simulink model "Prop_VV_jonny"  (R2020b)
settings: Solver=VariableStepAuto  StartTime=0.0  StopTime=10.0  RelTol=1e-3
settings Model: Creator=Jonathan van Zyl  LastModifiedBy=Jonathan van Zyl

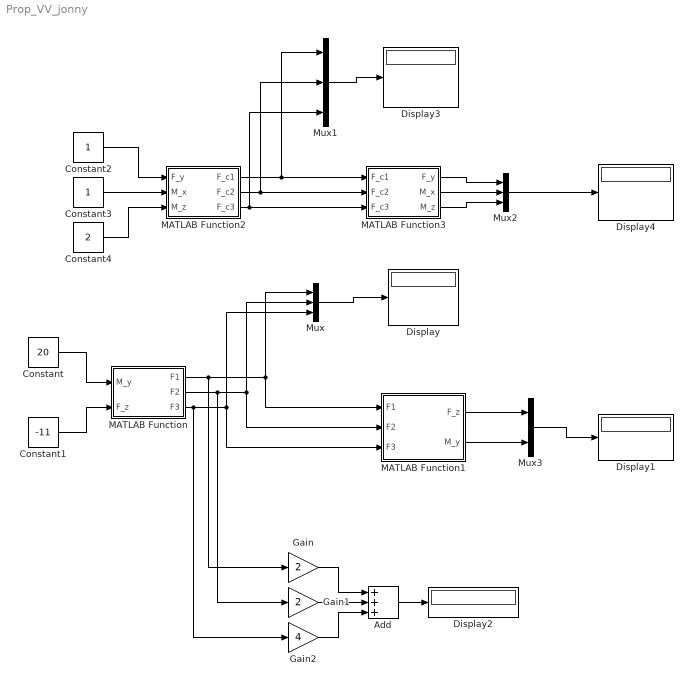
== system Prop_VV_jonny ==
  Add : Sum  Inputs=+++
  Constant : Constant  Value=20
  Constant1 : Constant  Value=-11
  Constant2 : Constant
  Constant3 : Constant
  Constant4 : Constant  Value=2
  Display{,1..4} (5 alike) : Display
  Gain : Gain  Gain=2
  Gain1 : Gain  Gain=2
  Gain2 : Gain  Gain=4
  MATLAB Function : MATLAB Function  TreatAsAtomicUnit=on
  MATLAB Function1 : MATLAB Function  TreatAsAtomicUnit=on
  MATLAB Function2 : MATLAB Function  TreatAsAtomicUnit=on
  MATLAB Function3 : MATLAB Function  TreatAsAtomicUnit=on
  Mux : Mux  Inputs=3
  Mux1 : Mux  Inputs=3
  Mux2 : Mux  Inputs=3
  Mux3 : Mux  Inputs=2
  wires:
  Constant/1 -> MATLAB Function/1(M_y)
  Constant1/1 -> MATLAB Function/2(F_z)
  MATLAB Function/1(F1) -> Gain/1, MATLAB Function1/1(F1), Mux/1
  MATLAB Function/2(F2) -> Gain1/1, MATLAB Function1/2(F2), Mux/2
  MATLAB Function/3(F3) -> Gain2/1, MATLAB Function1/3(F3), Mux/3
  Mux/1 -> Display/1
  Constant2/1 -> MATLAB Function2/1(F_y)
  Constant3/1 -> MATLAB Function2/2(M_x)
  Constant4/1 -> MATLAB Function2/3(M_z)
  MATLAB Function2/1(F_c1) -> MATLAB Function3/1(F_c1), Mux1/1
  MATLAB Function2/2(F_c2) -> MATLAB Function3/2(F_c2), Mux1/2
  MATLAB Function2/3(F_c3) -> Mux1/3, MATLAB Function3/3(F_c3)
  Mux1/1 -> Display3/1
  MATLAB Function3/1(F_y) -> Mux2/1
  MATLAB Function3/3(M_z) -> Mux2/3
  MATLAB Function3/2(M_x) -> Mux2/2
  Mux2/1 -> Display4/1
  MATLAB Function1/1(F_z) -> Mux3/1
  MATLAB Function1/2(M_y) -> Mux3/2
  Mux3/1 -> Display1/1
  Gain/1 -> Add/1
  Gain1/1 -> Add/2
  Gain2/1 -> Add/3
  Add/1 -> Display2/1

== matlab function Prop_VV_jonny/MATLAB Function1 ==
  data: F1 input; F_z output; F2 input; M_y output; F3 input
function [F_z, M_y] = fcn(F1, F2, F3)
xt_1 = 1.2598;
xb_1 = 2.2598;
xt_3 = -1.3402;
x_t1 = xt_1;
x_b1 = xb_1;
x_t3 = xt_3;

M_y = -100;
F_z = 0;

A_mat = [1 1;
    xt_1 xb_1];

A_inv = inv(A_mat);

force = [F1; F2];

back = A_mat*force;
backtrack = [4*F3; 4*F3*xt_3];
forceback = back+backtrack;
F_z = forceback(1);
M_y = forceback(2);
end

== matlab function Prop_VV_jonny/MATLAB Function ==
  data: M_y input; F1 output; F_z input; F2 output; F3 output
function [F1, F2, F3] = fcn(M_y, F_z)
xt_1 = 1.2598;
xb_1 = 2.2598;
xt_3 = -1.3402;
x_t1 = xt_1;
x_b1 = xb_1;
x_t3 = xt_3;



A_mat = [1 1;
    xt_1 xb_1];

A_inv = inv(A_mat);

p_0 = 0.2;
p_minus1 = 0;
step = 1000;
Converged = 0;
p_list = [];
x_list = [];
y_list = [];
J_list = [];
Fzz =[];
Myy =[];
while Converged == 0
    B = [(F_z - 4*p_0); (M_y - 4*p_0*xt_3)];
    force_0 = (A_inv*B);
    J_0 = sqrt(force_0(1)^2 + force_0(2)^2 + p_0^2);
    back = A_mat*force_0;
    backtrack = [4*p_0; 4*p_0*xt_3];
    forceback = back+backtrack;
    diff = sum(abs(forceback - [F_z; M_y]));
    if diff > 10^(-7)
        disp('Error')
        break
    end
    force = force_0;
    J = J_0;
    p = p_0;
    
    p_1 = p_0 + step;
    B = [(F_z - 4*p_1); (M_y - 4*p_1*xt_3)];
    force_1 = (A_inv*B);
    J_1 = sqrt(force_1(1)^2 + force_1(2)^2 + p_1^2);
    back = A_mat*force_1;
    backtrack = [4*p_1; 4*p_1*xt_3];
    forceback = back+backtrack;
    diff = sum(abs(forceback - [F_z; M_y]));
    if diff > 10^(-7)
        disp('Error')
        break
    end
    if J_1 < J_0
        force = force_1;
        J = J_1;
        p = p_1;
    end
    
    p_2 = p_0 - step;
    B = [(F_z - 4*p_2); (M_y - 4*p_2*xt_3)];
    force_2 = (A_inv*B);
    J_2 = sqrt(force_2(1)^2 + force_2(2)^2 + p_2^2);
    back = A_mat*force_2;
    backtrack = [4*p_2; 4*p_2*xt_3];
    forceback = back+backtrack;
    diff = sum(abs(forceback - [F_z; M_y]));
    if diff > 10^(-7)
        disp('Error')
        break
    end
    if J_2 < J_0 && J_2 < J_1
        force = force_2;
        J = J_2;
        p = p_2;
    end
    
    if p_minus1 < p_0 && p_0 < p
        step = step;
    elseif p_minus1 > p_0 && p_0 > p
        step = step;
    else
        step = step*0.9;
    end
        
    p_minus1 = p_0;
    p_0 = p;
    p_list = [p_list; p_0];
    x_list = [x_list; force(1)];
    y_list = [y_list; force(2)];
    J_list = [J_list; J];
    if step < abs(min([F_z,M_y])*10^(-9))
        Converged = 1;
    end
    
    
end

F1 = x_list(length(x_list));
F2 = y_list(length(y_list));
F3 = p_0;
end

== matlab function Prop_VV_jonny/MATLAB Function2 ==
  data: F_y input; F_c1 output; M_x input; M_z input; F_c2 output; F_c3 output
function [F_c1, F_c2, F_c3] = fcn(F_y, M_x, M_z)
%CATIA trans
TcgCatia = [1 0 0;
    0 -1 0;
    0 0 -1];

%Propeller arms - changed due to CATIA errors
c_1 = [-640.1998; 0; 506.566]*10^(-3);      %Control Back Top
c_2 = [-1040.1998; 0; -493.434]*10^(-3);    %Control Back Bottom
c_3 = [2259.8002; 0; -293.434]*10^(-3);     %Control Front

%Propeller arms - rotated
c_1 = TcgCatia*c_1;
c1 = transpose(c_1);
c_2 = TcgCatia*c_2;
c2 = transpose(c_2);
c_3 = TcgCatia*c_3;
c3 = transpose(c_3);

xc_1 = c1(1);
zc_1 = c1(3);

xc_2 = c2(1);
zc_2 = c2(3);

xc_3 = c3(1);
zc_3 = c3(3);

A_control = [1 1 1;
    zc_1 zc_2 zc_3;
    xc_1 xc_2 xc_3];
A_cinv = inv(A_control);
force_control = [F_y; M_x; M_z];
controlvec = A_cinv*force_control;
F_c1 = controlvec(1);
F_c2 = controlvec(2);
F_c3 = controlvec(3);
end

== matlab function Prop_VV_jonny/MATLAB Function3 ==
  data: F_c1 input; F_y output; M_x output; F_c2 input; F_c3 input; M_z output
function [F_y, M_x, M_z] = fcn(F_c1, F_c2, F_c3)

%CATIA trans
TcgCatia = [1 0 0;
    0 -1 0;
    0 0 -1];

%Propeller arms - changed due to CATIA errors
c_1 = [-640.1998; 0; 506.566]*10^(-3);      %Control Back Top
c_2 = [-1040.1998; 0; -493.434]*10^(-3);    %Control Back Bottom
c_3 = [2259.8002; 0; -293.434]*10^(-3);     %Control Front

%Propeller arms - rotated
c_1 = TcgCatia*c_1;
c1 = transpose(c_1);
c_2 = TcgCatia*c_2;
c2 = transpose(c_2);
c_3 = TcgCatia*c_3;
c3 = transpose(c_3);

xc_1 = c1(1);
zc_1 = c1(3);

xc_2 = c2(1);
zc_2 = c2(3);

xc_3 = c3(1);
zc_3 = c3(3);


Control_forces = [F_c1; F_c2; F_c3];

A_control = [1 1 1;
        zc_1 zc_2 zc_3;
        xc_1 xc_2 xc_3]; 
Control_vec_2 = A_control*Control_forces;
F_y = Control_vec_2(1);
M_x = Control_vec_2(2);
M_z = Control_vec_2(3);
end
